simulink model "rwa_allocation_test"  (R2018b)
settings: Solver=VariableStepAuto  StartTime=0.0  StopTime=60  RelTol=1e-3
undefined symbols (not defined in the file or in its folder): DiscIntNeverNeededParam
libraries: sharedutil x2, pd_control_lib x1, dynamics_lib x1, command_processing x1, reaction_wheel_assembly_lib x1
settings Model: Creator=Taylor  LastModifiedBy=Taylor

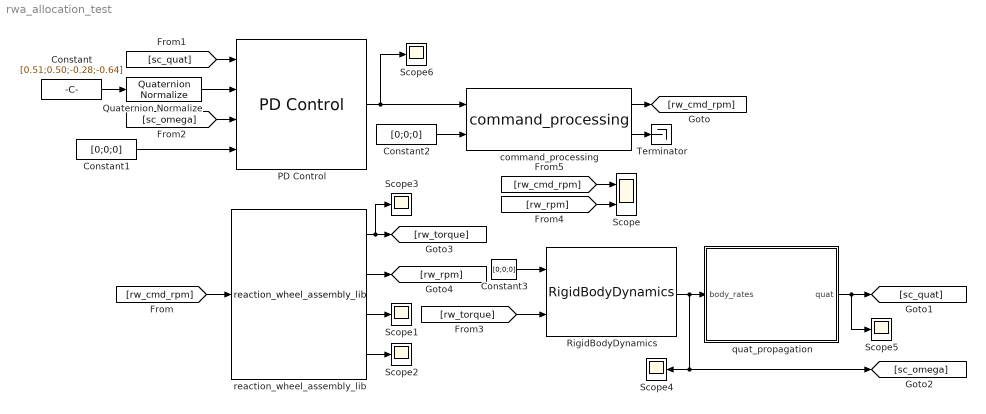
== system rwa_allocation_test ==
  Constant : Constant  Value=[0.51;0.50;-0.28;-0.64]
  Constant1 : Constant  Value=[0;0;0]
  Constant2 : Constant  Value=[0;0;0]
  Constant3 : Constant  Value=[0;0;0]
  PD Control : pd_control_lib/PD Control  SystemSampleTime=-1
  Quaternion Normalize : sharedutil/Quaternion Normalize  aMode=aMode
      settings: SourceProductName=Aerospace Blockset  SourceProductBaseCode=AE
  RigidBodyDynamics : dynamics_lib/Dynamics/RigidBodyDynamics  SystemSampleTime=-1
  Scope : Scope  NumInputPorts=2
  Scope{1..6} (6 alike) : Scope
  Terminator : Terminator
  command_processing : command_processing/command_processing  SystemSampleTime=-1
  quat_propagation : Subsystem  AncestorBlock=dynamics_lib/Dynamics/quat_propagation
  reaction_wheel_assembly_lib : reaction_wheel_assembly_lib/reaction_wheel_assembly_lib  SystemSampleTime=-1
  wires:
  PD Control/1 -> command_processing/1, Scope6/1
  Constant1/1 -> PD Control/4
  Constant/1 -> Quaternion Normalize/1
  RigidBodyDynamics/1 -> [sc_omega], Scope4/1, quat_propagation/1(body_rates)
  Constant2/1 -> command_processing/2
  command_processing/2 -> Terminator/1
  command_processing/1 -> [rw_cmd_rpm]
  [rw_cmd_rpm] -> reaction_wheel_assembly_lib/1
  reaction_wheel_assembly_lib/1 -> Scope3/1, [rw_torque]
  Constant3/1 -> RigidBodyDynamics/1
  quat_propagation/1(quat) -> Scope5/1, [sc_quat]
  [sc_quat] -> PD Control/1
  [sc_omega] -> PD Control/3
  reaction_wheel_assembly_lib/4 -> Scope2/1
  [rw_torque] -> RigidBodyDynamics/2
  reaction_wheel_assembly_lib/3 -> Scope1/1
  reaction_wheel_assembly_lib/2 -> [rw_rpm]
  [rw_rpm] -> Scope/2
  [rw_cmd_rpm] -> Scope/1
  Quaternion Normalize/1 -> PD Control/2

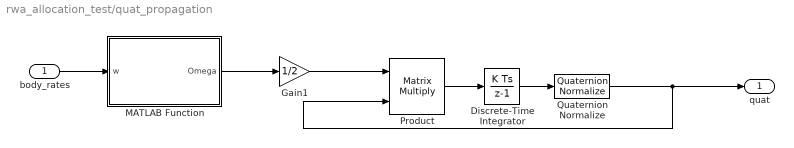
== system rwa_allocation_test/quat_propagation ==
  body_rates : Inport
  Discrete-Time Integrator : DiscreteIntegrator  InitialCondition=[0.831605;0.035124;0.004882;-0.554234]  SampleTime=-1  ICPrevOutput=DiscIntNeverNeededParam  ICPrevScaledInput=DiscIntNeverNeededParam
  Gain1 : Gain  Gain=1/2
  MATLAB Function : MATLAB Function  TreatAsAtomicUnit=on
  Product : Product  Multiplication=Matrix(*)  RndMeth=Zero
  Quaternion Normalize : sharedutil/Quaternion Normalize  aMode=aMode
      settings: SourceProductName=Aerospace Blockset  SourceProductBaseCode=AE
  quat : Outport
  wires:
  MATLAB Function/1(Omega) -> Gain1/1
  body_rates/1 -> MATLAB Function/1(w)
  Quaternion Normalize/1 -> Product/2, quat/1
  Gain1/1 -> Product/1
  Discrete-Time Integrator/1 -> Quaternion Normalize/1
  Product/1 -> Discrete-Time Integrator/1

== matlab function rwa_allocation_test/quat_propagation/MATLAB Function ==
  data: w input; Omega output
function Omega = skew_sym(w)
%#codegen

    w_skew = ...
        [0 w(3) -w(2);
        -w(3) 0 w(1);
        w(2) -w(1) 0];

    Omega = ...
        [0 -w';
        w w_skew];
